simulink model "Generico"  (R2016a)
settings: Solver=VariableStepAuto  StartTime=0.0  StopTime=10.0  RelTol=1e-3
values from neighbouring files (symbols this model uses):
  A = flip(fliplr(A))    [Guia.m]
  B = flip(B)    [Guia.m]
  C = fliplr(C)    [Guia.m]
  D = [0]    [Guia.m]
  Init_cond = zeros(1,size(A,1))    [Guia.m]
settings Model: Creator=adrie  LastModifiedBy=adrie
settings GRTTargetCC: GeneratePreprocessorConditionals=Use local settings

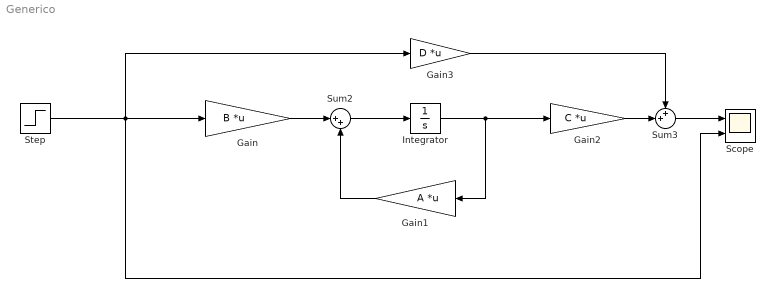
== system Generico ==
  Gain : Gain  Gain=B  Multiplication=Matrix(K*u) (u vector)
  Gain1 : Gain  Gain=A  Multiplication=Matrix(K*u) (u vector)
  Gain2 : Gain  Gain=C  Multiplication=Matrix(K*u) (u vector)
  Gain3 : Gain  Gain=D  Multiplication=Matrix(K*u) (u vector)
  Integrator : Integrator  InitialCondition=Init_cond
  Scope : Scope  NumInputPorts=2
  Step : Step  SampleTime=0
  Sum2 : Sum  Inputs=|++
  Sum3 : Sum  Inputs=++|
  wires:
  Gain/1 -> Sum2/1
  Sum2/1 -> Integrator/1
  Gain1/1 -> Sum2/2
  Integrator/1 -> Gain2/1, Gain1/1
  Gain2/1 -> Sum3/2
  Gain3/1 -> Sum3/1
  Sum3/1 -> Scope/1
  Step/1 -> Scope/2, Gain3/1, Gain/1
